simulink model "PID_control"  (R2018b)
settings: Solver=VariableStepAuto  StartTime=0.0  StopTime=10.0  RelTol=1e-3
values from neighbouring files (symbols this model uses):
  B = zeros(5,6)    [kalmanfilter.m]    (also in model_2017.m = [[0      0      0      0     ];                        [0   ; model_rough.m; model_v2.m = [[0      0      0      0     ];                        [0   ; model_v3.m = [[0      0      0      0      0      0             ];       )
  B_inv = pinv(B)    [kalmanfilter.m]    (also in model_rough.m)
  B_tx = -0.3    [model_rough.m]
  B_tz = -0.3    [model_rough.m]
  B_x = -0.3    [model_rough.m]
  B_y = -0.3    [model_rough.m]
  B_z = -0.3    [model_rough.m]
  I_x = Ix    [kalmanfilter.m]    (also in model_rough.m = parameters(2))
  I_z = Iz    [kalmanfilter.m]    (also in model_rough.m = parameters(4))
  M_x = m + Ma_x    [model_rough.m]
  M_y = m + Ma_y    [model_rough.m]
  M_z = m + Ma_z    [model_rough.m]
libraries: simulink x5
settings Model: Creator=Carter  LastModifiedBy=carter
settings SFSimCC: SimUseLocalCustomCode=off
settings RTWCC: RTWUseLocalCustomCode=off

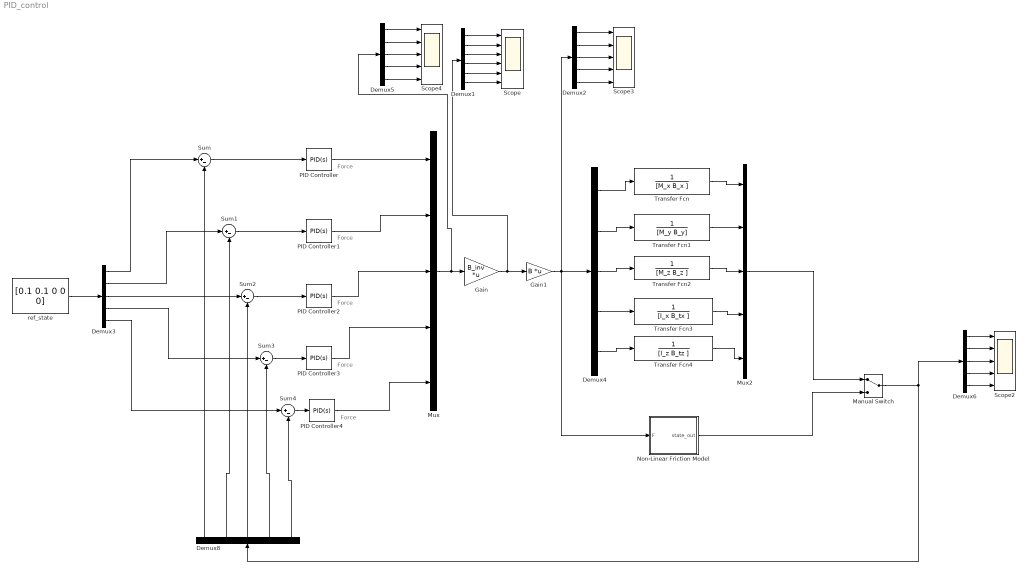
== system PID_control ==
  note: Force
  note: Force
  note: Force
  note: Force
  note: Force
  Demux1 : Demux  Outputs=6
  Demux{2..6,8} (6 alike) : Demux  Outputs=5
  Gain : Gain  Gain=B_inv  Multiplication=Matrix(K*u)
  Gain1 : Gain  Gain=B  Multiplication=Matrix(K*u)
  Manual Switch : ManualSwitch
  Mux : Mux  Inputs=5
  Mux2 : Mux  Inputs=5
  Non-Linear Friction Model : Subsystem
  PID Controller : simulink/Continuous/PID Controller  Controller=PID  Form=Parallel  TimeDomain=Continuous-time  SampleTime=-1  IntegratorMethod=Forward Euler  FilterMethod=Forward Euler  ControllerParametersSource=internal  P=300  I=0.5  D=9  UseFilter=on  N=0.0569750135499571  TunerSelectOption=Transfer Function Based (PID Tuner App)  InitialConditionSource=internal  InitialConditionForIntegrator=0  InitialConditionForFilter=0  DifferentiatorICPrevScaledInput=0  ExternalReset=none  TrackingMode=off  Kt=1  LimitOutput=off  UpperSaturationLimit=inf  LowerSaturationLimit=-inf  LinearizeAsGain=on  AntiWindupMode=none  Kb=1  POutMin=[]  POutMax=[]  IOutMin=[]  IOutMax=[]  DOutMin=[]  DOutMax=[]  NOutMin=[]  NOutMax=[]  SumOutMin=[]  SumOutMax=[]  SaturationOutMin=[]  SaturationOutMax=[]  PParamMin=[]  PParamMax=[]  IParamMin=[]  IParamMax=[]  DParamMin=[]  DParamMax=[]  NParamMin=[]  NParamMax=[]  KbParamMin=[]  KbParamMax=[]  KtParamMin=[]  KtParamMax=[]  KbOutMin=[]  KbOutMax=[]  KtOutMin=[]  KtOutMax=[]  IntegratorOutMin=[]  IntegratorOutMax=[]  FilterOutMin=[]  FilterOutMax=[]  SumI1OutMin=[]  SumI1OutMax=[]  SumI2OutMin=[]  SumI2OutMax=[]  SumI3OutMin=[]  SumI3OutMax=[]  SumI4OutMin=[]  SumI4OutMax=[]  SumDOutMin=[]  SumDOutMax=[]  DifferentiatorOutMin=[]  DifferentiatorOutMax=[]  FilterDiffOutCoefMin=[]  FilterDiffOutCoefMax=[]  ReciprocalOutMin=[]  ReciprocalOutMax=[]  SumDenOutMin=[]  SumDenOutMax=[]  SumNumOutMin=[]  SumNumOutMax=[]  DivideOutMin=[]  DivideOutMax=[]  IntegratorContinuousStateAttributes=''  IntegratorStateMustResolveToSignalObject=off  IntegratorRTWStateStorageClass=Auto  FilterContinuousStateAttributes=''  FilterStateMustResolveToSignalObject=off  FilterRTWStateStorageClass=Auto  ParallelPVariant=InternalParameters  IdealPVariant=Disabled  IVariant=InternalParameters  DVariant=InternalParameters  IntegratorVariant=Continuous  SatVariant=Disabled  AWVariant=Passthrough  PCopyVariant=Disabled  TRVariant=Disabled  FdbkBlocksVariant=Forward  IdealPFdbkVariant=Disabled  SatFdbkVariant=Disabled  DerivativeFilterVariant=ContFilter  NVariant=InternalParameters  NCopyVariant=Disabled  FilterICVariant=InternalICsFilter  IntegratorICVariant=InternalICs  ExternalResetVariant=Disabled  TRSumVariant=Passthrough  SumFdbkVariant=Disabled  SumVariant=Sum_PID
  PID Controller1 : simulink/Continuous/PID Controller  Controller=PID  Form=Parallel  TimeDomain=Continuous-time  SampleTime=-1  IntegratorMethod=Forward Euler  FilterMethod=Forward Euler  ControllerParametersSource=internal  P=300  I=0.5  D=0  UseFilter=on  N=0.0969723091680407  TunerSelectOption=Transfer Function Based (PID Tuner App)  InitialConditionSource=internal  InitialConditionForIntegrator=0  InitialConditionForFilter=0  DifferentiatorICPrevScaledInput=0  ExternalReset=none  TrackingMode=off  Kt=1  LimitOutput=off  UpperSaturationLimit=inf  LowerSaturationLimit=-inf  LinearizeAsGain=on  AntiWindupMode=none  Kb=1  POutMin=[]  POutMax=[]  IOutMin=[]  IOutMax=[]  DOutMin=[]  DOutMax=[]  NOutMin=[]  NOutMax=[]  SumOutMin=[]  SumOutMax=[]  SaturationOutMin=[]  SaturationOutMax=[]  PParamMin=[]  PParamMax=[]  IParamMin=[]  IParamMax=[]  DParamMin=[]  DParamMax=[]  NParamMin=[]  NParamMax=[]  KbParamMin=[]  KbParamMax=[]  KtParamMin=[]  KtParamMax=[]  KbOutMin=[]  KbOutMax=[]  KtOutMin=[]  KtOutMax=[]  IntegratorOutMin=[]  IntegratorOutMax=[]  FilterOutMin=[]  FilterOutMax=[]  SumI1OutMin=[]  SumI1OutMax=[]  SumI2OutMin=[]  SumI2OutMax=[]  SumI3OutMin=[]  SumI3OutMax=[]  SumI4OutMin=[]  SumI4OutMax=[]  SumDOutMin=[]  SumDOutMax=[]  DifferentiatorOutMin=[]  DifferentiatorOutMax=[]  FilterDiffOutCoefMin=[]  FilterDiffOutCoefMax=[]  ReciprocalOutMin=[]  ReciprocalOutMax=[]  SumDenOutMin=[]  SumDenOutMax=[]  SumNumOutMin=[]  SumNumOutMax=[]  DivideOutMin=[]  DivideOutMax=[]  IntegratorContinuousStateAttributes=''  IntegratorStateMustResolveToSignalObject=off  IntegratorRTWStateStorageClass=Auto  FilterContinuousStateAttributes=''  FilterStateMustResolveToSignalObject=off  FilterRTWStateStorageClass=Auto  ParallelPVariant=InternalParameters  IdealPVariant=Disabled  IVariant=InternalParameters  DVariant=InternalParameters  IntegratorVariant=Continuous  SatVariant=Disabled  AWVariant=Passthrough  PCopyVariant=Disabled  TRVariant=Disabled  FdbkBlocksVariant=Forward  IdealPFdbkVariant=Disabled  SatFdbkVariant=Disabled  DerivativeFilterVariant=ContFilter  NVariant=InternalParameters  NCopyVariant=Disabled  FilterICVariant=InternalICsFilter  IntegratorICVariant=InternalICs  ExternalResetVariant=Disabled  TRSumVariant=Passthrough  SumFdbkVariant=Disabled  SumVariant=Sum_PID
  PID Controller2 : simulink/Continuous/PID Controller  Controller=PID  Form=Parallel  TimeDomain=Continuous-time  SampleTime=-1  IntegratorMethod=Forward Euler  FilterMethod=Forward Euler  ControllerParametersSource=internal  P=1000  I=5  D=0  UseFilter=on  N=100  TunerSelectOption=Transfer Function Based (PID Tuner App)  InitialConditionSource=internal  InitialConditionForIntegrator=0  InitialConditionForFilter=0  DifferentiatorICPrevScaledInput=0  ExternalReset=none  TrackingMode=off  Kt=1  LimitOutput=off  UpperSaturationLimit=inf  LowerSaturationLimit=-inf  LinearizeAsGain=on  AntiWindupMode=none  Kb=1  POutMin=[]  POutMax=[]  IOutMin=[]  IOutMax=[]  DOutMin=[]  DOutMax=[]  NOutMin=[]  NOutMax=[]  SumOutMin=[]  SumOutMax=[]  SaturationOutMin=[]  SaturationOutMax=[]  PParamMin=[]  PParamMax=[]  IParamMin=[]  IParamMax=[]  DParamMin=[]  DParamMax=[]  NParamMin=[]  NParamMax=[]  KbParamMin=[]  KbParamMax=[]  KtParamMin=[]  KtParamMax=[]  KbOutMin=[]  KbOutMax=[]  KtOutMin=[]  KtOutMax=[]  IntegratorOutMin=[]  IntegratorOutMax=[]  FilterOutMin=[]  FilterOutMax=[]  SumI1OutMin=[]  SumI1OutMax=[]  SumI2OutMin=[]  SumI2OutMax=[]  SumI3OutMin=[]  SumI3OutMax=[]  SumI4OutMin=[]  SumI4OutMax=[]  SumDOutMin=[]  SumDOutMax=[]  DifferentiatorOutMin=[]  DifferentiatorOutMax=[]  FilterDiffOutCoefMin=[]  FilterDiffOutCoefMax=[]  ReciprocalOutMin=[]  ReciprocalOutMax=[]  SumDenOutMin=[]  SumDenOutMax=[]  SumNumOutMin=[]  SumNumOutMax=[]  DivideOutMin=[]  DivideOutMax=[]  IntegratorContinuousStateAttributes=''  IntegratorStateMustResolveToSignalObject=off  IntegratorRTWStateStorageClass=Auto  FilterContinuousStateAttributes=''  FilterStateMustResolveToSignalObject=off  FilterRTWStateStorageClass=Auto  ParallelPVariant=InternalParameters  IdealPVariant=Disabled  IVariant=InternalParameters  DVariant=InternalParameters  IntegratorVariant=Continuous  SatVariant=Disabled  AWVariant=Passthrough  PCopyVariant=Disabled  TRVariant=Disabled  FdbkBlocksVariant=Forward  IdealPFdbkVariant=Disabled  SatFdbkVariant=Disabled  DerivativeFilterVariant=ContFilter  NVariant=InternalParameters  NCopyVariant=Disabled  FilterICVariant=InternalICsFilter  IntegratorICVariant=InternalICs  ExternalResetVariant=Disabled  TRSumVariant=Passthrough  SumFdbkVariant=Disabled  SumVariant=Sum_PID
  PID Controller3 : simulink/Continuous/PID Controller  Controller=PID  Form=Parallel  TimeDomain=Continuous-time  SampleTime=-1  IntegratorMethod=Forward Euler  FilterMethod=Forward Euler  ControllerParametersSource=internal  P=1000  I=5  D=0  UseFilter=on  N=100  TunerSelectOption=Transfer Function Based (PID Tuner App)  InitialConditionSource=internal  InitialConditionForIntegrator=0  InitialConditionForFilter=0  DifferentiatorICPrevScaledInput=0  ExternalReset=none  TrackingMode=off  Kt=1  LimitOutput=off  UpperSaturationLimit=inf  LowerSaturationLimit=-inf  LinearizeAsGain=on  AntiWindupMode=none  Kb=1  POutMin=[]  POutMax=[]  IOutMin=[]  IOutMax=[]  DOutMin=[]  DOutMax=[]  NOutMin=[]  NOutMax=[]  SumOutMin=[]  SumOutMax=[]  SaturationOutMin=[]  SaturationOutMax=[]  PParamMin=[]  PParamMax=[]  IParamMin=[]  IParamMax=[]  DParamMin=[]  DParamMax=[]  NParamMin=[]  NParamMax=[]  KbParamMin=[]  KbParamMax=[]  KtParamMin=[]  KtParamMax=[]  KbOutMin=[]  KbOutMax=[]  KtOutMin=[]  KtOutMax=[]  IntegratorOutMin=[]  IntegratorOutMax=[]  FilterOutMin=[]  FilterOutMax=[]  SumI1OutMin=[]  SumI1OutMax=[]  SumI2OutMin=[]  SumI2OutMax=[]  SumI3OutMin=[]  SumI3OutMax=[]  SumI4OutMin=[]  SumI4OutMax=[]  SumDOutMin=[]  SumDOutMax=[]  DifferentiatorOutMin=[]  DifferentiatorOutMax=[]  FilterDiffOutCoefMin=[]  FilterDiffOutCoefMax=[]  ReciprocalOutMin=[]  ReciprocalOutMax=[]  SumDenOutMin=[]  SumDenOutMax=[]  SumNumOutMin=[]  SumNumOutMax=[]  DivideOutMin=[]  DivideOutMax=[]  IntegratorContinuousStateAttributes=''  IntegratorStateMustResolveToSignalObject=off  IntegratorRTWStateStorageClass=Auto  FilterContinuousStateAttributes=''  FilterStateMustResolveToSignalObject=off  FilterRTWStateStorageClass=Auto  ParallelPVariant=InternalParameters  IdealPVariant=Disabled  IVariant=InternalParameters  DVariant=InternalParameters  IntegratorVariant=Continuous  SatVariant=Disabled  AWVariant=Passthrough  PCopyVariant=Disabled  TRVariant=Disabled  FdbkBlocksVariant=Forward  IdealPFdbkVariant=Disabled  SatFdbkVariant=Disabled  DerivativeFilterVariant=ContFilter  NVariant=InternalParameters  NCopyVariant=Disabled  FilterICVariant=InternalICsFilter  IntegratorICVariant=InternalICs  ExternalResetVariant=Disabled  TRSumVariant=Passthrough  SumFdbkVariant=Disabled  SumVariant=Sum_PID
  PID Controller4 : simulink/Continuous/PID Controller  Controller=PID  Form=Parallel  TimeDomain=Continuous-time  SampleTime=-1  IntegratorMethod=Forward Euler  FilterMethod=Forward Euler  ControllerParametersSource=internal  P=1000  I=5  D=0  UseFilter=on  N=100  TunerSelectOption=Transfer Function Based (PID Tuner App)  InitialConditionSource=internal  InitialConditionForIntegrator=0  InitialConditionForFilter=0  DifferentiatorICPrevScaledInput=0  ExternalReset=none  TrackingMode=off  Kt=1  LimitOutput=off  UpperSaturationLimit=inf  LowerSaturationLimit=-inf  LinearizeAsGain=on  AntiWindupMode=none  Kb=1  POutMin=[]  POutMax=[]  IOutMin=[]  IOutMax=[]  DOutMin=[]  DOutMax=[]  NOutMin=[]  NOutMax=[]  SumOutMin=[]  SumOutMax=[]  SaturationOutMin=[]  SaturationOutMax=[]  PParamMin=[]  PParamMax=[]  IParamMin=[]  IParamMax=[]  DParamMin=[]  DParamMax=[]  NParamMin=[]  NParamMax=[]  KbParamMin=[]  KbParamMax=[]  KtParamMin=[]  KtParamMax=[]  KbOutMin=[]  KbOutMax=[]  KtOutMin=[]  KtOutMax=[]  IntegratorOutMin=[]  IntegratorOutMax=[]  FilterOutMin=[]  FilterOutMax=[]  SumI1OutMin=[]  SumI1OutMax=[]  SumI2OutMin=[]  SumI2OutMax=[]  SumI3OutMin=[]  SumI3OutMax=[]  SumI4OutMin=[]  SumI4OutMax=[]  SumDOutMin=[]  SumDOutMax=[]  DifferentiatorOutMin=[]  DifferentiatorOutMax=[]  FilterDiffOutCoefMin=[]  FilterDiffOutCoefMax=[]  ReciprocalOutMin=[]  ReciprocalOutMax=[]  SumDenOutMin=[]  SumDenOutMax=[]  SumNumOutMin=[]  SumNumOutMax=[]  DivideOutMin=[]  DivideOutMax=[]  IntegratorContinuousStateAttributes=''  IntegratorStateMustResolveToSignalObject=off  IntegratorRTWStateStorageClass=Auto  FilterContinuousStateAttributes=''  FilterStateMustResolveToSignalObject=off  FilterRTWStateStorageClass=Auto  ParallelPVariant=InternalParameters  IdealPVariant=Disabled  IVariant=InternalParameters  DVariant=InternalParameters  IntegratorVariant=Continuous  SatVariant=Disabled  AWVariant=Passthrough  PCopyVariant=Disabled  TRVariant=Disabled  FdbkBlocksVariant=Forward  IdealPFdbkVariant=Disabled  SatFdbkVariant=Disabled  DerivativeFilterVariant=ContFilter  NVariant=InternalParameters  NCopyVariant=Disabled  FilterICVariant=InternalICsFilter  IntegratorICVariant=InternalICs  ExternalResetVariant=Disabled  TRSumVariant=Passthrough  SumFdbkVariant=Disabled  SumVariant=Sum_PID
  Scope : Scope  NumInputPorts=6
  Scope2 : Scope  NumInputPorts=5
  Scope3 : Scope  NumInputPorts=5
  Scope4 : Scope  NumInputPorts=5
  Sum{,1..4} (5 alike) : Sum  Inputs=|+-
  Transfer Fcn : TransferFcn  Denominator=[M_x B_x ]
  Transfer Fcn1 : TransferFcn  Denominator=[M_y B_y]
  Transfer Fcn2 : TransferFcn  Denominator=[M_z B_z ]
  Transfer Fcn3 : TransferFcn  Denominator=[I_x B_tx ]
  Transfer Fcn4 : TransferFcn  Denominator=[I_z B_tz ]
  ref_state : Constant  Value=[0.1 0.1 0 0 0]
  wires:
  Demux3/1 -> Sum/1
  Sum/1 -> PID Controller/1
  Demux1/1 -> Scope/1
  Demux1/2 -> Scope/2
  Demux1/3 -> Scope/3
  Demux1/4 -> Scope/4
  Demux1/5 -> Scope/5
  Demux1/6 -> Scope/6
  Demux2/1 -> Scope3/1
  Demux2/3 -> Scope3/3
  Demux2/4 -> Scope3/4
  Demux2/5 -> Scope3/5
  Demux2/2 -> Scope3/2
  Sum1/1 -> PID Controller1/1
  Demux3/2 -> Sum1/1
  Sum2/1 -> PID Controller2/1
  Demux3/3 -> Sum2/1
  PID Controller3/1 -> Mux/4
  Sum3/1 -> PID Controller3/1
  Demux3/4 -> Sum3/1
  Sum4/1 -> PID Controller4/1
  Demux3/5 -> Sum4/1
  ref_state/1 -> Demux3/1
  PID Controller/1 -> Mux/1
  PID Controller1/1 -> Mux/2
  PID Controller2/1 -> Mux/3
  PID Controller4/1 -> Mux/5
  Gain/1 -> Demux1/1, Gain1/1
  Demux4/3 -> Transfer Fcn2/1
  Demux4/1 -> Transfer Fcn/1
  Demux4/2 -> Transfer Fcn1/1
  Demux4/4 -> Transfer Fcn3/1
  Demux4/5 -> Transfer Fcn4/1
  Demux5/3 -> Scope4/3
  Demux5/4 -> Scope4/4
  Demux5/5 -> Scope4/5
  Mux/1 -> Demux5/1, Gain/1
  Demux5/1 -> Scope4/1
  Demux5/2 -> Scope4/2
  Gain1/1 -> Non-Linear Friction Model/1(F), Demux2/1, Demux4/1
  Demux6/1 -> Scope2/1
  Demux6/2 -> Scope2/2
  Demux6/3 -> Scope2/3
  Demux6/4 -> Scope2/4
  Demux6/5 -> Scope2/5
  Transfer Fcn/1 -> Mux2/1
  Transfer Fcn1/1 -> Mux2/2
  Transfer Fcn2/1 -> Mux2/3
  Transfer Fcn3/1 -> Mux2/4
  Transfer Fcn4/1 -> Mux2/5
  Non-Linear Friction Model/1(state_out) -> Manual Switch/2
  Mux2/1 -> Manual Switch/1
  Demux8/1 -> Sum/2
  Demux8/2 -> Sum1/2
  Demux8/3 -> Sum2/2
  Demux8/4 -> Sum3/2
  Demux8/5 -> Sum4/2
  Manual Switch/1 -> Demux6/1, Demux8/1

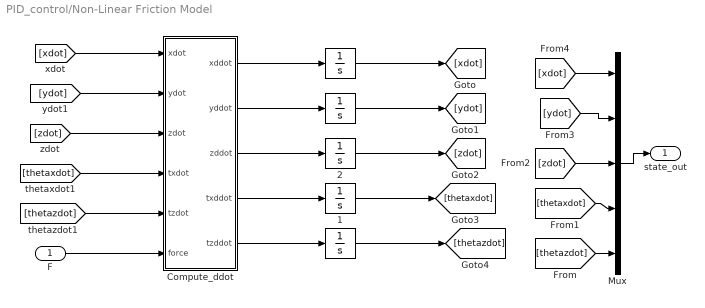
== system PID_control/Non-Linear Friction Model ==
  F : Inport
  "  " : Integrator
  "   " : Integrator
  "    " : Integrator
  "  1" : Integrator
  "  2" : Integrator
  Compute_ddot : MATLAB Function  TreatAsAtomicUnit=on
  Mux : Mux  Inputs=5
  state_out : Outport
  wires:
  F/1 -> Compute_ddot/6(force)
  [thetaxdot] -> Compute_ddot/4(txdot)
  [zdot] -> Compute_ddot/3(zdot)
  [ydot] -> Compute_ddot/2(ydot)
  Compute_ddot/2(yddot) -> "    "/1
  [xdot] -> Compute_ddot/1(xdot)
  Mux/1 -> state_out/1
  [thetazdot] -> Compute_ddot/5(tzdot)
  Compute_ddot/5(tzddot) -> "  "/1
  Compute_ddot/1(xddot) -> "   "/1
  Compute_ddot/4(txddot) -> "  1"/1
  Compute_ddot/3(zddot) -> "  2"/1
  "   "/1 -> [xdot]
  "    "/1 -> [ydot]
  "  2"/1 -> [zdot]
  "  1"/1 -> [thetaxdot]
  "  "/1 -> [thetazdot]
  [thetazdot] -> Mux/5
  [thetaxdot] -> Mux/4
  [zdot] -> Mux/3
  [ydot] -> Mux/2
  [xdot] -> Mux/1

== matlab function PID_control/Non-Linear Friction Model/Compute_ddot ==
  data: xddot output; xdot input; ydot input; yddot output; zdot input; txdot input; tzdot input; zddot output; txddot output; tzddot output; force input
function [xddot, yddot, zddot, txddot, tzddot] = get_ddot(xdot, ydot, zdot, txdot, tzdot, force)

% Load inertia, added inertia
m = 24.5;
ma_x = 12.8340;
ma_y = 17.3295;
ma_z = 21.9371;
I_x = 1.7047;
I_z = 1.6031;

% Load friction parameters and thruster matrix
% Friction = k_L*v + k_Q*v^2

% TEMP
k_Lx = 0;
k_Ly = 0;
k_Lz = 0;
k_Ltx = 0;
k_Ltz = 0;

k_Qx = 1.001076306811700e+02;
k_Qy = 85.738911664000000;
k_Qz = 1.081401140888600e+02;
k_Qtx = 1.081401140888600e+02;
k_Qtz = 85.738911664000000;

L_diags = 0.48; 
L_sides = 0.21;

B = zeros(5,6); 
B(1,:) = [cosd(45) cosd(45) cosd(45) cosd(45) 0 0];
B(2,:) = [cosd(45) -cosd(45) cosd(45) -cosd(45) 0 0];
B(3,:) = [ 0 0 0 0 1 1];
B(4,:) = [ 0 0 0 0 -L_sides L_sides];
B(5,:) = [-L_diags L_diags L_diags -L_diags 0 0];

% Standard for input u
% u = [F_sf, F_pf, F_sb, F_pb, F_st, F_pt]
% port, starboard, front, back, top

if(length(force) == 5)
    % Compute linear forces and torques F_x, F_y, F_z, T_x, T_z
    xddot = (force(1)- k_Lx*(xdot) -k_Qx*abs(xdot^2))/(m+ma_x);
    yddot = (force(2) - k_Ly*(ydot) -k_Qy*abs(ydot^2))/(m+ma_y);
    zddot = (force(3)- k_Lz*(zdot) -k_Qz*abs(zdot^2))/(m+ma_z);

    txddot = (force(4)- k_Ltx*(txdot) -k_Qtx*abs(txdot^2))/I_x;
    tzddot = (force(5)- k_Ltz*(tzdot) -k_Qtz*abs(tzdot^2))/I_z;
else
    xddot = 0;
    yddot = 0;
    zddot = 0;
    
    txddot = 0;
    tzddot = 0;
end
